simulink model "prescribed_time_ES"  (R2024a)
settings: Solver=FixedStepAuto  StartTime=0.0  StopTime=5  FixedStep=0.0001  RelTol=1e-3
values from neighbouring files (symbols this model uses):
  a = 0.05    [prescribed_time_parameters.m]    (also in unbiased_ES_parameters.m)
  k = 0.005    [prescribed_time_parameters.m]    (also in unbiased_ES_parameters.m)
  lambda = 0.05    [prescribed_time_parameters.m]    (also in unbiased_ES_parameters.m)
  T = 5.3    [prescribed_time_parameters.m]
  w = 5    [prescribed_time_parameters.m]    (also in unbiased_ES_parameters.m)
  wh = 3    [prescribed_time_parameters.m]    (also in unbiased_ES_parameters.m)
undefined symbols (not defined in the file or in its folder): National_Instruments, PCI
libraries: cstblocks x3, sldrtlib x2
settings Model: SimulationMode=external  ExtModeTrigDuration=50001  ExtModeArchiveMode=auto  ExtModeArchiveFileName=seeking_data  ExtModeArchiveDirName=C:\Users\Eric\nonlinear-adaptive-control-lab-extremum-seeking-photovoltaic-experiment\data\12-8-perscribed-data\perscribed  ExtModeLogAll=off  Creator=CTY  LastModifiedBy=Eric
settings HardwareCC: ProdBitPerLong=64  ProdHWDeviceType=Intel->x86-64 (Linux 64)
settings ModelReferenceCC: EnableRefExpFcnMdlSchedulingChecks=on
settings RTWCC: Description=Simulink Desktop Real-Time  SystemTargetFile=sldrt.tlc  TemplateMakefile=sldrt.tmf  TargetLang=C++  RTWCompilerOptimization=on  GPUComputeCapability=3.5
settings CodeAppCC: MaxIdLength=95
settings SimulinkDesktopRealTimeCC: TargetLibSuffix=_sldrt.a  TargetPreCompLibLocation=C:\Program Files\MATLAB\R2024a\toolbox\sldrt\lib\win64  TargetLangStandard=C++11 (ISO)

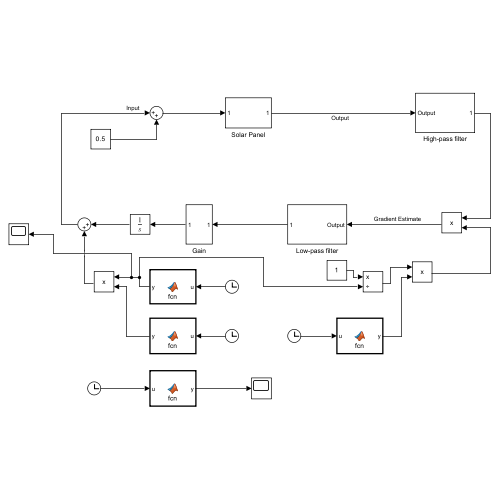
[thumbnail: Simulink's stored preview of the top-level diagram]
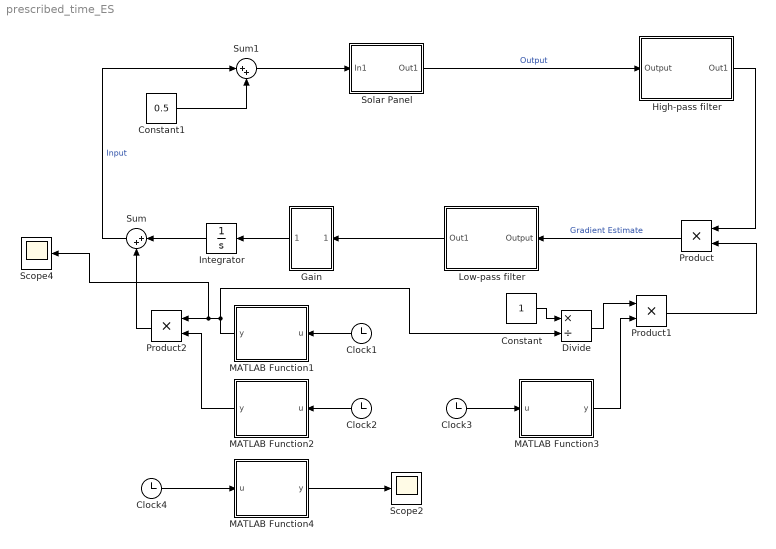
== system prescribed_time_ES ==
  Clock{1..4} (4 alike) : Clock
  Constant : Constant
  Constant1 : Constant  Value=0.5
  Divide : Product  Inputs=*/
  Gain : Subsystem
  High-pass filter : Subsystem
  Integrator : Integrator
  Low-pass filter : Subsystem
  MATLAB Function1 : MATLAB Function  TreatAsAtomicUnit=on
  MATLAB Function2 : MATLAB Function  TreatAsAtomicUnit=on
  MATLAB Function3 : MATLAB Function  TreatAsAtomicUnit=on
  MATLAB Function4 : MATLAB Function  TreatAsAtomicUnit=on
  Product : Product
  Product1 : Product
  Product2 : Product
  Scope2 : Scope
  Scope4 : Scope
  Solar Panel : Subsystem
  Sum : Sum  Inputs=|++
  Sum1 : Sum  Inputs=|++
  wires:
  Solar Panel/1(Out1) -> High-pass filter/1(Output)  "Output"
  Product/1 -> Low-pass filter/1(Output)  "Gradient Estimate"
  Product1/1 -> Product/2
  Product2/1 -> Sum/2
  MATLAB Function2/1(y) -> Product2/2
  MATLAB Function3/1(y) -> Product1/2
  MATLAB Function1/1(y) -> Divide/2, Scope4/1, Product2/1
  Constant/1 -> Divide/1
  Divide/1 -> Product1/1
  High-pass filter/1(Out1) -> Product/1
  Low-pass filter/1(Out1) -> Gain/1(In1)
  Clock1/1 -> MATLAB Function1/1(u)
  Clock2/1 -> MATLAB Function2/1(u)
  Clock3/1 -> MATLAB Function3/1(u)
  Integrator/1 -> Sum/1
  Gain/1(Out1) -> Integrator/1
  MATLAB Function4/1(y) -> Scope2/1
  Clock4/1 -> MATLAB Function4/1(u)
  Sum1/1 -> Solar Panel/1(In1)
  Sum/1 -> Sum1/1  "Input"
  Constant1/1 -> Sum1/2

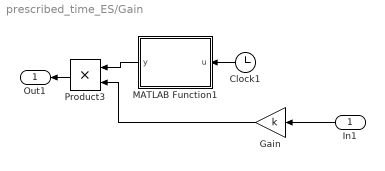
== system prescribed_time_ES/Gain ==
  In1 : Inport
  Clock1 : Clock
  Gain : Gain  Gain=k
  MATLAB Function1 : MATLAB Function  TreatAsAtomicUnit=on
  Product3 : Product
  Out1 : Outport
  wires:
  MATLAB Function1/1(y) -> Product3/1
  Clock1/1 -> MATLAB Function1/1(u)
  Gain/1 -> Product3/2
  In1/1 -> Gain/1
  Product3/1 -> Out1/1

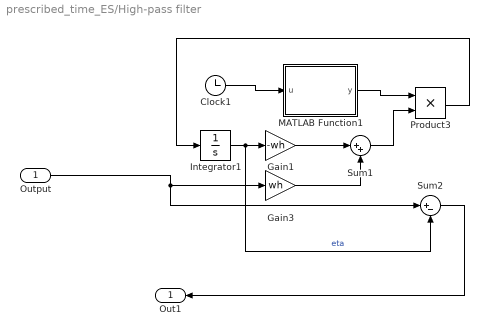
== system prescribed_time_ES/High-pass filter ==
  Output : Inport
  Clock1 : Clock
  Gain1 : Gain  Gain=-wh
  Gain3 : Gain  Gain=wh
  Integrator1 : Integrator
  MATLAB Function1 : MATLAB Function  TreatAsAtomicUnit=on
  Product3 : Product
  Sum1 : Sum  Inputs=|++
  Sum2 : Sum  Inputs=|+-
  Out1 : Outport
  wires:
  Integrator1/1 -> Sum2/2, Gain1/1  "eta"
  Product3/1 -> Integrator1/1
  Gain1/1 -> Sum1/1
  MATLAB Function1/1(y) -> Product3/1
  Clock1/1 -> MATLAB Function1/1(u)
  Sum1/1 -> Product3/2
  Output/1 -> Sum2/1, Gain3/1
  Gain3/1 -> Sum1/2
  Sum2/1 -> Out1/1

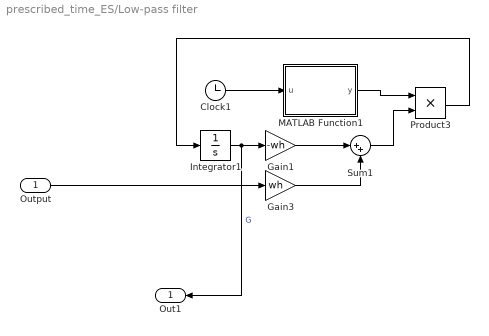
== system prescribed_time_ES/Low-pass filter ==
  Output : Inport
  Clock1 : Clock
  Gain1 : Gain  Gain=-wh
  Gain3 : Gain  Gain=wh
  Integrator1 : Integrator
  MATLAB Function1 : MATLAB Function  TreatAsAtomicUnit=on
  Product3 : Product
  Sum1 : Sum  Inputs=|++
  Out1 : Outport
  wires:
  Integrator1/1 -> Out1/1, Gain1/1  "G"
  Product3/1 -> Integrator1/1
  Gain1/1 -> Sum1/1
  MATLAB Function1/1(y) -> Product3/1
  Clock1/1 -> MATLAB Function1/1(u)
  Sum1/1 -> Product3/2
  Output/1 -> Gain3/1
  Gain3/1 -> Sum1/2

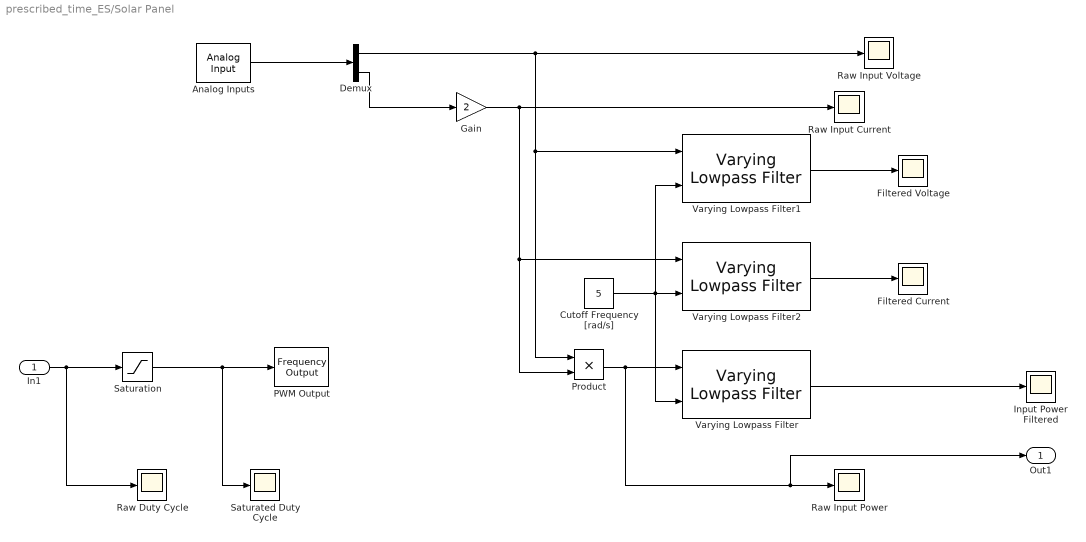
== system prescribed_time_ES/Solar Panel ==
  In1 : Inport
  Analog Inputs : sldrtlib/Analog Input  SampleTime=0.001  MaxMissedTicks=100  ShowMissedTicks=off  YieldWhenWaiting=off  DrvName=National_Instruments/PCI-6251  DrvAddress=4294967295  DrvOptions=[1 0 0 3 3]  Channels=[1, 2]  RangeMode=1  VoltRange=1  DataType=1
      settings: AttributesFormatString=National Instruments\nPCI-6251 [auto]
  Cutoff Frequency [rad/s] : Constant  Value=5
  Demux : Demux  Outputs=2
  Filtered Current : Scope
  Filtered Voltage : Scope
  Gain : Gain  Gain=2
  Input Power Filtered : Scope
  PWM Output : sldrtlib/Frequency Output  SampleTime=0.0001  MaxMissedTicks=100000  ShowMissedTicks=off  YieldWhenWaiting=off  DrvName=National_Instruments/PCI-6251  DrvAddress=4294967295  DrvOptions=[1 0 0 3 3]  Channels=1  FrequencySource=1  Frequency=200000  FrequencyFinalValue=[]  DutySource=2  Duty=[]  DutyFinalValue=[]
      settings: AttributesFormatString=National Instruments\nPCI-6251 [auto]
  Product : Product
  Raw Duty Cycle : Scope
  Raw Input Current : Scope
  Raw Input Power : Scope
  Raw Input Voltage : Scope
  Saturated Duty Cycle : Scope
  Saturation : Saturate  UpperLimit=0.9  LowerLimit=0.2
  Varying Lowpass Filter : cstblocks/Linear Parameter Varying/Varying Lowpass Filter  N=1
  Varying Lowpass Filter1 : cstblocks/Linear Parameter Varying/Varying Lowpass Filter  N=1
  Varying Lowpass Filter2 : cstblocks/Linear Parameter Varying/Varying Lowpass Filter  N=1
  Out1 : Outport
  wires:
  Gain/1 -> Raw Input Current/1, Varying Lowpass Filter2/1, Product/2
  Analog Inputs/1 -> Demux/1
  In1/1 -> Raw Duty Cycle/1, Saturation/1
  Demux/2 -> Gain/1
  Demux/1 -> Raw Input Voltage/1, Varying Lowpass Filter1/1, Product/1
  Varying Lowpass Filter2/1 -> Filtered Current/1
  Cutoff Frequency [rad/s]/1 -> Varying Lowpass Filter1/2, Varying Lowpass Filter2/2, Varying Lowpass Filter/2
  Varying Lowpass Filter1/1 -> Filtered Voltage/1
  Varying Lowpass Filter/1 -> Input Power Filtered/1
  Saturation/1 -> Saturated Duty Cycle/1, PWM Output/1
  Product/1 -> Out1/1, Raw Input Power/1, Varying Lowpass Filter/1

== matlab function prescribed_time_ES/High-pass filter/MATLAB Function1 ==
  data: u input; y output; T parameter
function y = fcn(u, T)

y = T/(T-u);

== matlab function prescribed_time_ES/Low-pass filter/MATLAB Function1 ==
  data: u input; y output; T parameter
function y = fcn(u, T)

y = T/(T-u);

== matlab function prescribed_time_ES/Gain/MATLAB Function1 ==
  data: u input; y output; T parameter
function y = fcn(u, T)

y = T/(T-u);

== matlab function prescribed_time_ES/MATLAB Function1 ==
  data: u input; y output; lambda parameter; T parameter
function y = fcn(u, lambda, T)

y = (T/(T-u))^(-lambda*T);

== matlab function prescribed_time_ES/MATLAB Function2 ==
  data: u input; y output; a parameter; T parameter; w parameter
function y = fcn(u, a, T, w)

y = a*sin(w*T*log(T/(T-u)));

== matlab function prescribed_time_ES/MATLAB Function3 ==
  data: u input; y output; a parameter; w parameter; T parameter
function y = fcn(u, a, w, T)

y = 2/a*sin(w*T*log(T/(T-u)));

== matlab function prescribed_time_ES/MATLAB Function4 ==
  data: u input; y output; a parameter; T parameter; w parameter
function y = fcn(u, a, T, w)

y = w*T^2/(T-u)^2;
